simulink model "Serial_to_sample"  (R2017a)
settings: Solver=VariableStepAuto  StartTime=0.0  StopTime=inf  RelTol=1e-3
libraries: dspindex x1, instrumentlib x1
settings Model: Creator=LuisFernando  LastModifiedBy=LuisFernando

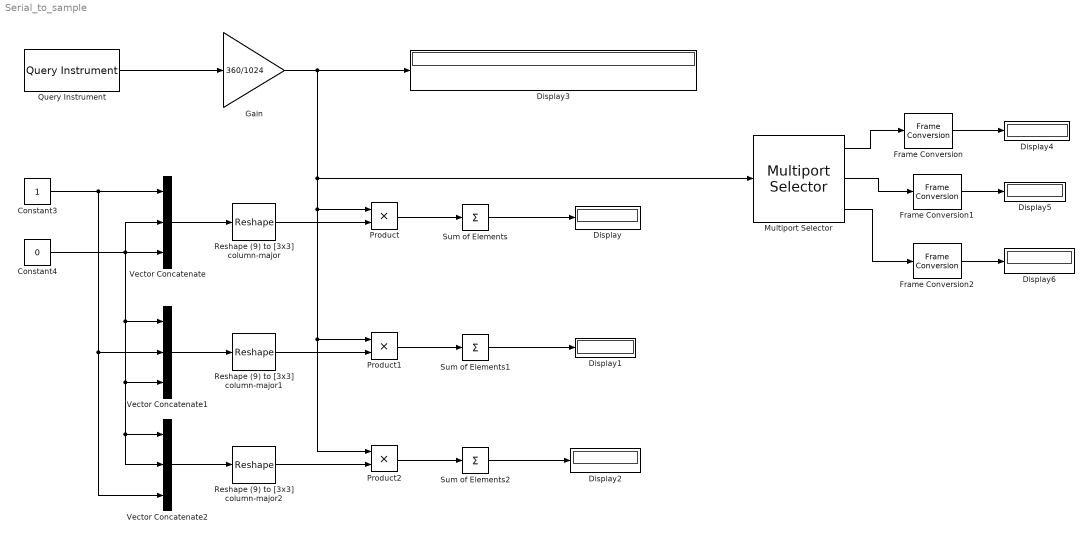
== system Serial_to_sample ==
  Constant3 : Constant
  Constant4 : Constant  Value=0
  Display{,1..6} (7 alike) : Display
  Frame Conversion : FrameConversion  InheritSamplingMode=off  OutFrame=Sample-based
  Frame Conversion1 : FrameConversion  InheritSamplingMode=off  OutFrame=Sample-based
  Frame Conversion2 : FrameConversion  InheritSamplingMode=off  OutFrame=Sample-based
  Gain : Gain  Gain=360/1024
  Multiport Selector : dspindex/Multiport Selector  rowsOrCols=Rows  idxCellArray={1,2,3}  idxErrMode=Clip Index
  Product : Product
  Product1 : Product
  Product2 : Product
  Query Instrument : instrumentlib/Query Instrument  sampleTime=100  isWorkspaceObject=off  timeout=2  inputBufferSize=1000  protocol=Serial  serialPort=COM4  baudRate=9600  gpibVendor=Agilent Technologies  boardIndex=0  primaryAddress=1  secondaryAddress=0  visaVendor=Agilent  visaSerialPort=0  chassisIndex=0  logicalAddress=0  tcpRemoteHost='127.0.0.1'  tcpRemotePort=4500  udpRemoteHost='127.0.0.1'  udpRemotePort=9090  visaTCPBoardIndex=0  visaTCPRemoteHost='127.0.0.1'  usbBoardIndex=0  usbManufID=0  usbModelCode=0  usbSerialNumber=0  wsVariableName=puerto  initAction=None  initCommand='DATA:SOURCE CH1'  initFunction=get  queryCommand='1r'  responseFormat=ASCII  asciiFormatting=',%d,%d,%dr'  precision=8-bit integer  byteOrder=Little endian  valuesToRead=1  removeBytes=off  afterOutputAction=Repeat query for new data  enableFrames=on  frameSize=3
      settings: SourceProductName=Instrument Control Toolbox  SourceProductBaseCode=IC
  Reshape (9) to [3x3] column-major : Reshape  OutputDimensionality=Column vector (2-D)  OutputDimensions=[1,3]
  Reshape (9) to [3x3] column-major1 : Reshape  OutputDimensionality=Column vector (2-D)  OutputDimensions=[1,3]
  Reshape (9) to [3x3] column-major2 : Reshape  OutputDimensionality=Column vector (2-D)  OutputDimensions=[1,3]
  Sum of Elements : Sum  Inputs=+
  Sum of Elements1 : Sum  Inputs=+
  Sum of Elements2 : Sum  Inputs=+
  Vector Concatenate : Concatenate  NumInputs=3
  Vector Concatenate1 : Concatenate  NumInputs=3
  Vector Concatenate2 : Concatenate  NumInputs=3
  wires:
  Sum of Elements1/1 -> Display1/1
  Gain/1 -> Multiport Selector/1, Product1/1, Product2/1, Product/1, Display3/1
  Constant4/1 -> Vector Concatenate2/1, Vector Concatenate2/2, Vector Concatenate1/3, Vector Concatenate1/1, Vector Concatenate/2, Vector Concatenate/3
  Sum of Elements/1 -> Display/1
  Product2/1 -> Sum of Elements2/1
  Vector Concatenate1/1 -> Reshape (9) to [3x3] column-major1/1
  Query Instrument/1 -> Gain/1
  Vector Concatenate2/1 -> Reshape (9) to [3x3] column-major2/1
  Sum of Elements2/1 -> Display2/1
  Reshape (9) to [3x3] column-major1/1 -> Product1/2
  Product1/1 -> Sum of Elements1/1
  Vector Concatenate/1 -> Reshape (9) to [3x3] column-major/1
  Reshape (9) to [3x3] column-major/1 -> Product/2
  Constant3/1 -> Vector Concatenate2/3, Vector Concatenate1/2, Vector Concatenate/1
  Product/1 -> Sum of Elements/1
  Reshape (9) to [3x3] column-major2/1 -> Product2/2
  Multiport Selector/1 -> Frame Conversion/1
  Frame Conversion/1 -> Display4/1
  Frame Conversion1/1 -> Display5/1
  Multiport Selector/2 -> Frame Conversion1/1
  Multiport Selector/3 -> Frame Conversion2/1
  Frame Conversion2/1 -> Display6/1
